simulink model "lab_3_task_2_a_simulink"  (R2025b)
settings: Solver=VariableStepAuto  StartTime=0.0  StopTime=10.0  RelTol=1e-3
values from neighbouring files (symbols this model uses):
  I = diag([ix iy iz])    [lab_3_task_3.m]    (also in lab_4_task_3.m; lab_5_task_1.m; lab_5_task_2.m; lab_6_task_1.m = diag([ ix iy iz ]))
undefined symbols (not defined in the file or in its folder): I_a, w_a
libraries: matrix_library x1
settings Model: Creator=User  LastModifiedBy=User

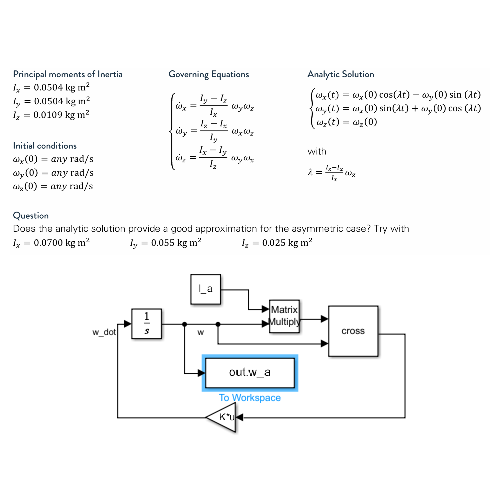
[thumbnail: Simulink's stored preview of the top-level diagram]
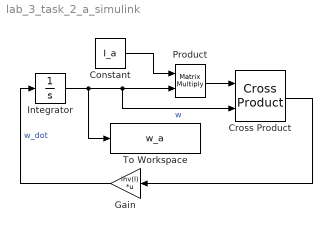
== system lab_3_task_2_a_simulink ==
  Constant : Constant  Value=I_a
  Cross Product : matrix_library/Cross Product
  Gain : Gain  Gain=inv(I)  Multiplication=Matrix(K*u)
  Integrator : Integrator  InitialCondition=w_a
  Product : Product  Multiplication=Matrix(*)
  To Workspace : ToWorkspace  VariableName=w_a  SaveFormat=Timeseries  SampleTime=-1
  wires:
  Product/1 -> Cross Product/1
  Gain/1 -> Integrator/1  "w_dot"
  Constant/1 -> Product/1
  Integrator/1 -> To Workspace/1, Cross Product/2, Product/2  "w"
  Cross Product/1 -> Gain/1
